simulink model "math_pendulum_model"  (R2021b)
settings: Solver=VariableStepAuto  StartTime=0.0  StopTime=10.0  MaxStep=0.05  RelTol=1e-3
libraries: simulink_extras x1
settings Model: Creator=USER  LastModifiedBy=USER

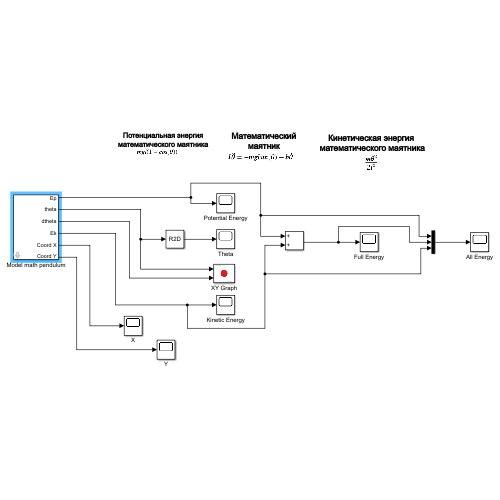
[thumbnail: Simulink's stored preview of the top-level diagram]
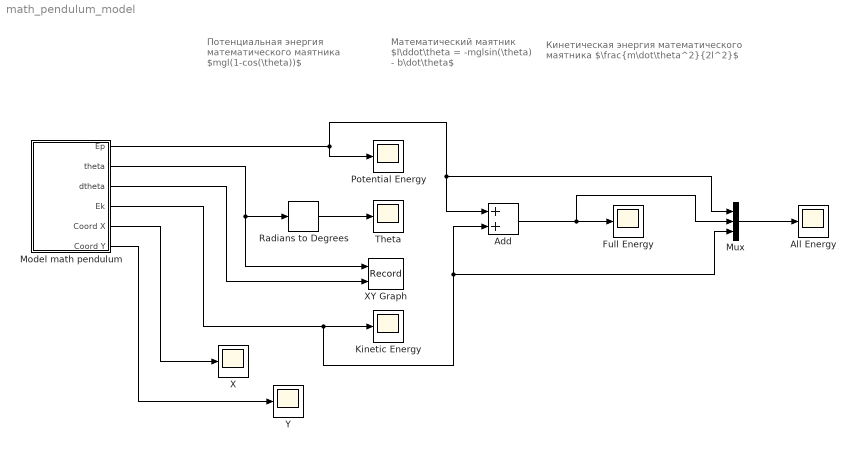
== system math_pendulum_model ==
  note: Кинетическая энергия
      | математического маятника
      | $\frac{m\dot\theta^2}{2l^2}$
  note: Потенциальная энергия математического маятника
      | $mgl(1-cos(\theta))$
  note: Математический маятник
      | $I\ddot\theta = -mglsin(\theta) - b\dot\theta$
  Add : Sum
  All Energy : Scope
  Full Energy : Scope
  Kinetic Energy : Scope
  Model math pendulum : Subsystem  mask{m=1, l=1, g=9.8, start_angle_deg=30, b=0.5}
      mask prompts: m "Mass"; l "Length"; g "Acceleration free downfall"; start_angle_deg "Start angle"; b "Dissipative member"
      mask init:
      | I = m * l^2
  Mux : Mux  Inputs=3
  Potential Energy : Scope
  Radians to Degrees : simulink_extras/Transformations/Radians to Degrees
  Theta : Scope
  X : Scope
  XY Graph : Record  FileSettingsInternal="{\"entries\":[{\"content\":{\"excelSettings\":{\"content\":{},\"type\":\"Streamout.ExcelSettings\"}},\"type\":\"Streamout.FileSettingStorage\",\"uuid\":\"6018c531-afb2-45bd-8a48-60115f8f832c\"}],\"packageUris\":[\"http://schema.mathworks.com/mf0/streamout_blocks/R2020a\"],\"version\":\"1.0\"}"  Layout=[1 1]  SignalsInternal="{\"entries\":[{\"content\":{\"signals\":[{\"content\":{\"blockPath\":[\"math_pendulum_model/XY Graph\"],\"channel\":[],\"dimensions\":[1],\"domain\":\"math_pendulum_model/XY Graph\",\"lineColor\":\"#a2142f\",\"plots\":[1],\"port\":1,\"sid\":[],\"signalID\":9,\"signalName\":\"Model math pendulum:2\"},\"type\":\"RecordBlkView.Signal\",\"uuid\":\"40beffd5-f63d-431c-b268-e8e84a637eab\"},{\"content\":{\"blockPath\":[\"math_pendulum_model/XY Graph\"],\"channel\":[],\"dimensions\":[1],\"domain\":\"math_pendulum_model/XY Graph\",\"lineColor\":\"#139fff\",\"plots\":[1],\"port\":2,\"sid\":[],\"signalID\":12,\"signalName\":\"Model math pendulum:3\"},\"type\":\"RecordBlkView.Signal\",\"uuid\":\"15e7a49c-6e59-4af3-aa91-2038b1727c98\"}]},\"type\":\"RecordBlkView.InputSignals\",\"uuid\":\"0d8cb8e2-806d-43b9-8564-6fa8db1dfa51\"}],\"packageUris\":[\"http://schema.mathworks.com/mf0/streamout_blocks/R2020a\"],\"version\":\"1.0\"}"  VisualizationBindings="{\"xyplotplugin\":{\"info\":[{\"series\":[{\"bindingParametersList\":[{\"parameter\":\"X-Axis\",\"signalID\":9,\"signalName\":\"Model math pendulum:2\"},{\"parameter\":\"Y-Axis\",\"signalID\":12,\"signalName\":\"Model math pendulum:3\"}],\"seriesID\":12590}],\"subplotID\":1}]}}"  CompatibilityTag=XY
  Y : Scope
  wires:
  Radians to Degrees/1 -> Theta/1
  Model math pendulum/2(theta) -> XY Graph/1, Radians to Degrees/1
  Model math pendulum/3(dtheta) -> XY Graph/2
  Add/1 -> Mux/2, Full Energy/1
  Mux/1 -> All Energy/1
  Model math pendulum/4(Ek) -> Mux/3, Add/2, Kinetic Energy/1
  Model math pendulum/1(Ep) -> Potential Energy/1, Mux/1, Add/1
  Model math pendulum/5(Coord X) -> X/1
  Model math pendulum/6(Coord Y) -> Y/1

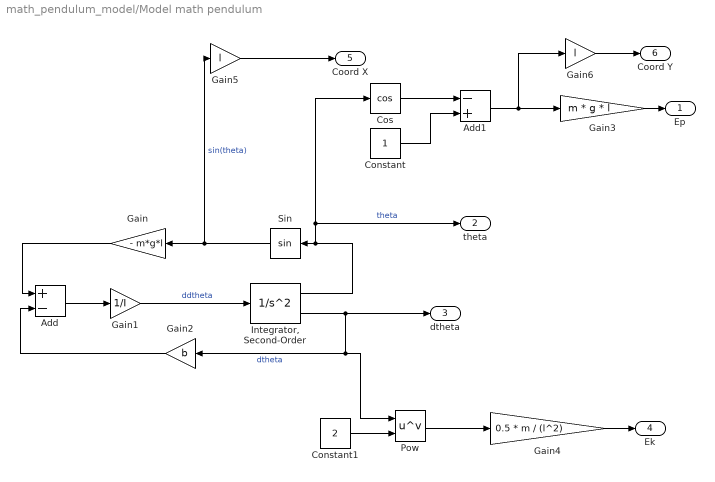
== system math_pendulum_model/Model math pendulum ==
  Add : Sum  Inputs=+-
  Add1 : Sum  Inputs=-+
  Constant : Constant
  Constant1 : Constant  Value=2
  Cos : Trigonometry  Operator=cos
  Gain : Gain  Gain=- m*g*l
  Gain1 : Gain  Gain=1/I
  Gain2 : Gain  Gain=b
  Gain3 : Gain  Gain=m * g * l
  Gain4 : Gain  Gain=0.5 * m / (l^2)
  Gain5 : Gain  Gain=l
  Gain6 : Gain  Gain=l
  "Integrator, Second-Order" : SecondOrderIntegrator  ICX=deg2rad(start_angle_deg)
  Pow : Math  Operator=pow  SignedPower=on  RndMeth=Zero  SaturateOnIntegerOverflow=on
  Sin : Trigonometry
  Ep : Outport
  theta : Outport  Port=2
  dtheta : Outport  Port=3
  Ek : Outport  Port=4
  Coord X : Outport  Port=5
  Coord Y : Outport  Port=6
  wires:
  Gain1/1 -> "Integrator, Second-Order"/1  "ddtheta"
  "Integrator, Second-Order"/2 -> Pow/1, Gain2/1, dtheta/1  "dtheta"
  Sin/1 -> Gain5/1, Gain/1  "sin(theta)"
  "Integrator, Second-Order"/1 -> Cos/1, theta/1, Sin/1  "theta"
  Gain/1 -> Add/1
  Gain2/1 -> Add/2
  Add/1 -> Gain1/1
  Gain3/1 -> Ep/1
  Add1/1 -> Gain6/1, Gain3/1
  Constant/1 -> Add1/2
  Pow/1 -> Gain4/1
  Gain4/1 -> Ek/1
  Constant1/1 -> Pow/2
  Gain5/1 -> Coord X/1
  Gain6/1 -> Coord Y/1
  Cos/1 -> Add1/1
